simulink model "SignalModel"  (R2017a)
settings: Solver=FixedStepAuto  StartTime=0.0  StopTime=10  FixedStep=0.01  RelTol=1e-3
libraries: simulink x3
settings Model: Creator=roman  LastModifiedBy=roman

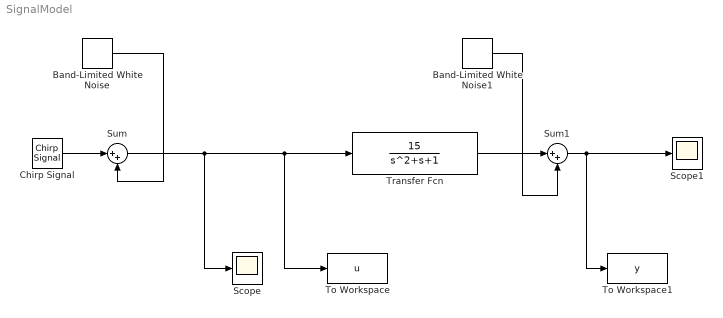
== system SignalModel ==
  Band-Limited White Noise : simulink/Sources/Band-Limited White Noise  Cov=[0.005]  Ts=0.1  seed=[23341]
  Band-Limited White Noise1 : simulink/Sources/Band-Limited White Noise  Cov=[0.0005]  Ts=0.05  seed=[23341]
  Chirp Signal : simulink/Sources/Chirp Signal  f1=0  T=10  f2=10
  Scope : Scope
  Scope1 : Scope
  Sum : Sum  Inputs=|++
  Sum1 : Sum  Inputs=|++
  To Workspace : ToWorkspace  VariableName=u  SampleTime=-1
  To Workspace1 : ToWorkspace  VariableName=y  SampleTime=-1
  Transfer Fcn : TransferFcn  Numerator=[15]  Denominator=[1 1 1]
  wires:
  Chirp Signal/1 -> Sum/1
  Band-Limited White Noise/1 -> Sum/2
  Sum/1 -> To Workspace/1, Transfer Fcn/1, Scope/1
  Band-Limited White Noise1/1 -> Sum1/2
  Transfer Fcn/1 -> Sum1/1
  Sum1/1 -> To Workspace1/1, Scope1/1
